simulink model "LV_grid"  (R2019b)
settings: Solver=VariableStepAuto  StartTime=0  StopTime=5.005  FixedStep=5e-4  RelTol=1e-3
model workspace (MAT data in the model file):
  P2_1 = 3450
libraries: powerlib x373, powerlib_meascontrol x37
(part 4 of 5)

== system LV_grid/L2/L1 ==
  Pi Section Line : powerlib/Elements/Pi Section Line  LConnTagsString=__new0  RConnTagsString=__new0  Frequency=50  Resistance=0.274  Inductance=0.073  Capacitance=12.74e-9  Length=0.0025  PiSections=1  Measurements=None
      settings: AttributesFormatString=\n  SourceProductName=Simscape Electrical  SourceProductBaseCode=PS
  Three-Phase PI Section Line : powerlib/Elements/Three-Phase PI Section Line  LConnTagsString=a|b|c  RConnTagsString=A|B|C  Frequency=50  Resistances=[ 0.274 0.959]  Inductances=[ 0.073 0.079]  Capacitances=[12.74e-9 7.751e-9]  Length=0.0025
      settings: SourceProductName=Simscape Electrical
  A : PMIOPort  Side=Left
  B : PMIOPort  Port=2  Side=Left
  C : PMIOPort  Port=3  Side=Left
  N : PMIOPort  Port=4  Side=Left
  a : PMIOPort  Port=5  Side=Right
  b : PMIOPort  Port=6  Side=Right
  c : PMIOPort  Port=7  Side=Right
  n : PMIOPort  Port=8  Side=Right
  connections:
  Pi Section Line/LConn1 -- N/RConn1
  Pi Section Line/RConn1 -- n/RConn1
  C/RConn1 -- Three-Phase PI Section Line/LConn3
  B/RConn1 -- Three-Phase PI Section Line/LConn2
  A/RConn1 -- Three-Phase PI Section Line/LConn1
  Three-Phase PI Section Line/RConn3 -- c/RConn1
  Three-Phase PI Section Line/RConn2 -- b/RConn1
  Three-Phase PI Section Line/RConn1 -- a/RConn1

== system LV_grid/L20/L1 ==
  Pi Section Line : powerlib/Elements/Pi Section Line  LConnTagsString=__new0  RConnTagsString=__new0  Frequency=50  Resistance=0.274  Inductance=0.073  Capacitance=12.74e-9  Length=0.0025  PiSections=1  Measurements=None
      settings: AttributesFormatString=\n  SourceProductName=Simscape Electrical  SourceProductBaseCode=PS
  Three-Phase PI Section Line : powerlib/Elements/Three-Phase PI Section Line  LConnTagsString=a|b|c  RConnTagsString=A|B|C  Frequency=50  Resistances=[ 0.274 0.959]  Inductances=[ 0.073 0.079]  Capacitances=[12.74e-9 7.751e-9]  Length=0.0025
      settings: SourceProductName=Simscape Electrical
  A : PMIOPort  Side=Left
  B : PMIOPort  Port=2  Side=Left
  C : PMIOPort  Port=3  Side=Left
  N : PMIOPort  Port=4  Side=Left
  a : PMIOPort  Port=5  Side=Right
  b : PMIOPort  Port=6  Side=Right
  c : PMIOPort  Port=7  Side=Right
  n : PMIOPort  Port=8  Side=Right
  connections:
  Pi Section Line/LConn1 -- N/RConn1
  Pi Section Line/RConn1 -- n/RConn1
  C/RConn1 -- Three-Phase PI Section Line/LConn3
  B/RConn1 -- Three-Phase PI Section Line/LConn2
  A/RConn1 -- Three-Phase PI Section Line/LConn1
  Three-Phase PI Section Line/RConn3 -- c/RConn1
  Three-Phase PI Section Line/RConn2 -- b/RConn1
  Three-Phase PI Section Line/RConn1 -- a/RConn1

== system LV_grid/L20/L2 ==
  Pi Section Line : powerlib/Elements/Pi Section Line  LConnTagsString=__new0  RConnTagsString=__new0  Frequency=50  Resistance=0.274  Inductance=0.073  Capacitance=12.74e-9  Length=0.0025  PiSections=1  Measurements=None
      settings: AttributesFormatString=\n  SourceProductName=Simscape Electrical  SourceProductBaseCode=PS
  Three-Phase PI Section Line : powerlib/Elements/Three-Phase PI Section Line  LConnTagsString=a|b|c  RConnTagsString=A|B|C  Frequency=50  Resistances=[ 0.274 0.959]  Inductances=[ 0.073 0.079]  Capacitances=[12.74e-9 7.751e-9]  Length=0.0025
      settings: SourceProductName=Simscape Electrical
  A : PMIOPort  Side=Left
  B : PMIOPort  Port=2  Side=Left
  C : PMIOPort  Port=3  Side=Left
  N : PMIOPort  Port=4  Side=Left
  a : PMIOPort  Port=5  Side=Right
  b : PMIOPort  Port=6  Side=Right
  c : PMIOPort  Port=7  Side=Right
  n : PMIOPort  Port=8  Side=Right
  connections:
  Pi Section Line/LConn1 -- N/RConn1
  Pi Section Line/RConn1 -- n/RConn1
  C/RConn1 -- Three-Phase PI Section Line/LConn3
  B/RConn1 -- Three-Phase PI Section Line/LConn2
  A/RConn1 -- Three-Phase PI Section Line/LConn1
  Three-Phase PI Section Line/RConn3 -- c/RConn1
  Three-Phase PI Section Line/RConn2 -- b/RConn1
  Three-Phase PI Section Line/RConn1 -- a/RConn1

== system LV_grid/L20/L3 ==
  Pi Section Line : powerlib/Elements/Pi Section Line  LConnTagsString=__new0  RConnTagsString=__new0  Frequency=50  Resistance=0.274  Inductance=0.073  Capacitance=12.74e-9  Length=0.0025  PiSections=1  Measurements=None
      settings: AttributesFormatString=\n  SourceProductName=Simscape Electrical  SourceProductBaseCode=PS
  Three-Phase PI Section Line : powerlib/Elements/Three-Phase PI Section Line  LConnTagsString=a|b|c  RConnTagsString=A|B|C  Frequency=50  Resistances=[ 0.274 0.959]  Inductances=[ 0.073 0.079]  Capacitances=[12.74e-9 7.751e-9]  Length=0.0025
      settings: SourceProductName=Simscape Electrical
  A : PMIOPort  Side=Left
  B : PMIOPort  Port=2  Side=Left
  C : PMIOPort  Port=3  Side=Left
  N : PMIOPort  Port=4  Side=Left
  a : PMIOPort  Port=5  Side=Right
  b : PMIOPort  Port=6  Side=Right
  c : PMIOPort  Port=7  Side=Right
  n : PMIOPort  Port=8  Side=Right
  connections:
  Pi Section Line/LConn1 -- N/RConn1
  Pi Section Line/RConn1 -- n/RConn1
  C/RConn1 -- Three-Phase PI Section Line/LConn3
  B/RConn1 -- Three-Phase PI Section Line/LConn2
  A/RConn1 -- Three-Phase PI Section Line/LConn1
  Three-Phase PI Section Line/RConn3 -- c/RConn1
  Three-Phase PI Section Line/RConn2 -- b/RConn1
  Three-Phase PI Section Line/RConn1 -- a/RConn1

== system LV_grid/L21/L1 ==
  Pi Section Line : powerlib/Elements/Pi Section Line  LConnTagsString=__new0  RConnTagsString=__new0  Frequency=50  Resistance=0.274  Inductance=0.073  Capacitance=12.74e-9  Length=0.0025  PiSections=1  Measurements=None
      settings: AttributesFormatString=\n  SourceProductName=Simscape Electrical  SourceProductBaseCode=PS
  Three-Phase PI Section Line : powerlib/Elements/Three-Phase PI Section Line  LConnTagsString=a|b|c  RConnTagsString=A|B|C  Frequency=50  Resistances=[ 0.274 0.959]  Inductances=[ 0.073 0.079]  Capacitances=[12.74e-9 7.751e-9]  Length=0.0025
      settings: SourceProductName=Simscape Electrical
  A : PMIOPort  Side=Left
  B : PMIOPort  Port=2  Side=Left
  C : PMIOPort  Port=3  Side=Left
  N : PMIOPort  Port=4  Side=Left
  a : PMIOPort  Port=5  Side=Right
  b : PMIOPort  Port=6  Side=Right
  c : PMIOPort  Port=7  Side=Right
  n : PMIOPort  Port=8  Side=Right
  connections:
  Pi Section Line/LConn1 -- N/RConn1
  Pi Section Line/RConn1 -- n/RConn1
  C/RConn1 -- Three-Phase PI Section Line/LConn3
  B/RConn1 -- Three-Phase PI Section Line/LConn2
  A/RConn1 -- Three-Phase PI Section Line/LConn1
  Three-Phase PI Section Line/RConn3 -- c/RConn1
  Three-Phase PI Section Line/RConn2 -- b/RConn1
  Three-Phase PI Section Line/RConn1 -- a/RConn1

== system LV_grid/L21/L2 ==
  Pi Section Line : powerlib/Elements/Pi Section Line  LConnTagsString=__new0  RConnTagsString=__new0  Frequency=50  Resistance=0.274  Inductance=0.073  Capacitance=12.74e-9  Length=0.0025  PiSections=1  Measurements=None
      settings: AttributesFormatString=\n  SourceProductName=Simscape Electrical  SourceProductBaseCode=PS
  Three-Phase PI Section Line : powerlib/Elements/Three-Phase PI Section Line  LConnTagsString=a|b|c  RConnTagsString=A|B|C  Frequency=50  Resistances=[ 0.274 0.959]  Inductances=[ 0.073 0.079]  Capacitances=[12.74e-9 7.751e-9]  Length=0.0025
      settings: SourceProductName=Simscape Electrical
  A : PMIOPort  Side=Left
  B : PMIOPort  Port=2  Side=Left
  C : PMIOPort  Port=3  Side=Left
  N : PMIOPort  Port=4  Side=Left
  a : PMIOPort  Port=5  Side=Right
  b : PMIOPort  Port=6  Side=Right
  c : PMIOPort  Port=7  Side=Right
  n : PMIOPort  Port=8  Side=Right
  connections:
  Pi Section Line/LConn1 -- N/RConn1
  Pi Section Line/RConn1 -- n/RConn1
  C/RConn1 -- Three-Phase PI Section Line/LConn3
  B/RConn1 -- Three-Phase PI Section Line/LConn2
  A/RConn1 -- Three-Phase PI Section Line/LConn1
  Three-Phase PI Section Line/RConn3 -- c/RConn1
  Three-Phase PI Section Line/RConn2 -- b/RConn1
  Three-Phase PI Section Line/RConn1 -- a/RConn1

== system LV_grid/L21/L3 ==
  Pi Section Line : powerlib/Elements/Pi Section Line  LConnTagsString=__new0  RConnTagsString=__new0  Frequency=50  Resistance=0.274  Inductance=0.073  Capacitance=12.74e-9  Length=0.0025  PiSections=1  Measurements=None
      settings: AttributesFormatString=\n  SourceProductName=Simscape Electrical  SourceProductBaseCode=PS
  Three-Phase PI Section Line : powerlib/Elements/Three-Phase PI Section Line  LConnTagsString=a|b|c  RConnTagsString=A|B|C  Frequency=50  Resistances=[ 0.274 0.959]  Inductances=[ 0.073 0.079]  Capacitances=[12.74e-9 7.751e-9]  Length=0.0025
      settings: SourceProductName=Simscape Electrical
  A : PMIOPort  Side=Left
  B : PMIOPort  Port=2  Side=Left
  C : PMIOPort  Port=3  Side=Left
  N : PMIOPort  Port=4  Side=Left
  a : PMIOPort  Port=5  Side=Right
  b : PMIOPort  Port=6  Side=Right
  c : PMIOPort  Port=7  Side=Right
  n : PMIOPort  Port=8  Side=Right
  connections:
  Pi Section Line/LConn1 -- N/RConn1
  Pi Section Line/RConn1 -- n/RConn1
  C/RConn1 -- Three-Phase PI Section Line/LConn3
  B/RConn1 -- Three-Phase PI Section Line/LConn2
  A/RConn1 -- Three-Phase PI Section Line/LConn1
  Three-Phase PI Section Line/RConn3 -- c/RConn1
  Three-Phase PI Section Line/RConn2 -- b/RConn1
  Three-Phase PI Section Line/RConn1 -- a/RConn1

== system LV_grid/L21/L4 ==
  Pi Section Line : powerlib/Elements/Pi Section Line  LConnTagsString=__new0  RConnTagsString=__new0  Frequency=50  Resistance=0.274  Inductance=0.073  Capacitance=12.74e-9  Length=0.0025  PiSections=1  Measurements=None
      settings: AttributesFormatString=\n  SourceProductName=Simscape Electrical  SourceProductBaseCode=PS
  Three-Phase PI Section Line : powerlib/Elements/Three-Phase PI Section Line  LConnTagsString=a|b|c  RConnTagsString=A|B|C  Frequency=50  Resistances=[ 0.274 0.959]  Inductances=[ 0.073 0.079]  Capacitances=[12.74e-9 7.751e-9]  Length=0.0025
      settings: SourceProductName=Simscape Electrical
  A : PMIOPort  Side=Left
  B : PMIOPort  Port=2  Side=Left
  C : PMIOPort  Port=3  Side=Left
  N : PMIOPort  Port=4  Side=Left
  a : PMIOPort  Port=5  Side=Right
  b : PMIOPort  Port=6  Side=Right
  c : PMIOPort  Port=7  Side=Right
  n : PMIOPort  Port=8  Side=Right
  connections:
  Pi Section Line/LConn1 -- N/RConn1
  Pi Section Line/RConn1 -- n/RConn1
  C/RConn1 -- Three-Phase PI Section Line/LConn3
  B/RConn1 -- Three-Phase PI Section Line/LConn2
  A/RConn1 -- Three-Phase PI Section Line/LConn1
  Three-Phase PI Section Line/RConn3 -- c/RConn1
  Three-Phase PI Section Line/RConn2 -- b/RConn1
  Three-Phase PI Section Line/RConn1 -- a/RConn1

== system LV_grid/L21/L5 ==
  Pi Section Line : powerlib/Elements/Pi Section Line  LConnTagsString=__new0  RConnTagsString=__new0  Frequency=50  Resistance=0.274  Inductance=0.073  Capacitance=12.74e-9  Length=0.0025  PiSections=1  Measurements=None
      settings: AttributesFormatString=\n  SourceProductName=Simscape Electrical  SourceProductBaseCode=PS
  Three-Phase PI Section Line : powerlib/Elements/Three-Phase PI Section Line  LConnTagsString=a|b|c  RConnTagsString=A|B|C  Frequency=50  Resistances=[ 0.274 0.959]  Inductances=[ 0.073 0.079]  Capacitances=[12.74e-9 7.751e-9]  Length=0.0025
      settings: SourceProductName=Simscape Electrical
  A : PMIOPort  Side=Left
  B : PMIOPort  Port=2  Side=Left
  C : PMIOPort  Port=3  Side=Left
  N : PMIOPort  Port=4  Side=Left
  a : PMIOPort  Port=5  Side=Right
  b : PMIOPort  Port=6  Side=Right
  c : PMIOPort  Port=7  Side=Right
  n : PMIOPort  Port=8  Side=Right
  connections:
  Pi Section Line/LConn1 -- N/RConn1
  Pi Section Line/RConn1 -- n/RConn1
  C/RConn1 -- Three-Phase PI Section Line/LConn3
  B/RConn1 -- Three-Phase PI Section Line/LConn2
  A/RConn1 -- Three-Phase PI Section Line/LConn1
  Three-Phase PI Section Line/RConn3 -- c/RConn1
  Three-Phase PI Section Line/RConn2 -- b/RConn1
  Three-Phase PI Section Line/RConn1 -- a/RConn1

== system LV_grid/L22/L1 ==
  Pi Section Line : powerlib/Elements/Pi Section Line  LConnTagsString=__new0  RConnTagsString=__new0  Frequency=50  Resistance=0.274  Inductance=0.073  Capacitance=12.74e-9  Length=0.0025  PiSections=1  Measurements=None
      settings: AttributesFormatString=\n  SourceProductName=Simscape Electrical  SourceProductBaseCode=PS
  Three-Phase PI Section Line : powerlib/Elements/Three-Phase PI Section Line  LConnTagsString=a|b|c  RConnTagsString=A|B|C  Frequency=50  Resistances=[ 0.274 0.959]  Inductances=[ 0.073 0.079]  Capacitances=[12.74e-9 7.751e-9]  Length=0.0025
      settings: SourceProductName=Simscape Electrical
  A : PMIOPort  Side=Left
  B : PMIOPort  Port=2  Side=Left
  C : PMIOPort  Port=3  Side=Left
  N : PMIOPort  Port=4  Side=Left
  a : PMIOPort  Port=5  Side=Right
  b : PMIOPort  Port=6  Side=Right
  c : PMIOPort  Port=7  Side=Right
  n : PMIOPort  Port=8  Side=Right
  connections:
  Pi Section Line/LConn1 -- N/RConn1
  Pi Section Line/RConn1 -- n/RConn1
  C/RConn1 -- Three-Phase PI Section Line/LConn3
  B/RConn1 -- Three-Phase PI Section Line/LConn2
  A/RConn1 -- Three-Phase PI Section Line/LConn1
  Three-Phase PI Section Line/RConn3 -- c/RConn1
  Three-Phase PI Section Line/RConn2 -- b/RConn1
  Three-Phase PI Section Line/RConn1 -- a/RConn1

== system LV_grid/L22/L2 ==
  Pi Section Line : powerlib/Elements/Pi Section Line  LConnTagsString=__new0  RConnTagsString=__new0  Frequency=50  Resistance=0.274  Inductance=0.073  Capacitance=12.74e-9  Length=0.0025  PiSections=1  Measurements=None
      settings: AttributesFormatString=\n  SourceProductName=Simscape Electrical  SourceProductBaseCode=PS
  Three-Phase PI Section Line : powerlib/Elements/Three-Phase PI Section Line  LConnTagsString=a|b|c  RConnTagsString=A|B|C  Frequency=50  Resistances=[ 0.274 0.959]  Inductances=[ 0.073 0.079]  Capacitances=[12.74e-9 7.751e-9]  Length=0.0025
      settings: SourceProductName=Simscape Electrical
  A : PMIOPort  Side=Left
  B : PMIOPort  Port=2  Side=Left
  C : PMIOPort  Port=3  Side=Left
  N : PMIOPort  Port=4  Side=Left
  a : PMIOPort  Port=5  Side=Right
  b : PMIOPort  Port=6  Side=Right
  c : PMIOPort  Port=7  Side=Right
  n : PMIOPort  Port=8  Side=Right
  connections:
  Pi Section Line/LConn1 -- N/RConn1
  Pi Section Line/RConn1 -- n/RConn1
  C/RConn1 -- Three-Phase PI Section Line/LConn3
  B/RConn1 -- Three-Phase PI Section Line/LConn2
  A/RConn1 -- Three-Phase PI Section Line/LConn1
  Three-Phase PI Section Line/RConn3 -- c/RConn1
  Three-Phase PI Section Line/RConn2 -- b/RConn1
  Three-Phase PI Section Line/RConn1 -- a/RConn1

== system LV_grid/L23/L1 ==
  Pi Section Line : powerlib/Elements/Pi Section Line  LConnTagsString=__new0  RConnTagsString=__new0  Frequency=50  Resistance=0.274  Inductance=0.073  Capacitance=12.74e-9  Length=0.0025  PiSections=1  Measurements=None
      settings: AttributesFormatString=\n  SourceProductName=Simscape Electrical  SourceProductBaseCode=PS
  Three-Phase PI Section Line : powerlib/Elements/Three-Phase PI Section Line  LConnTagsString=a|b|c  RConnTagsString=A|B|C  Frequency=50  Resistances=[ 0.274 0.959]  Inductances=[ 0.073 0.079]  Capacitances=[12.74e-9 7.751e-9]  Length=0.0025
      settings: SourceProductName=Simscape Electrical
  A : PMIOPort  Side=Left
  B : PMIOPort  Port=2  Side=Left
  C : PMIOPort  Port=3  Side=Left
  N : PMIOPort  Port=4  Side=Left
  a : PMIOPort  Port=5  Side=Right
  b : PMIOPort  Port=6  Side=Right
  c : PMIOPort  Port=7  Side=Right
  n : PMIOPort  Port=8  Side=Right
  connections:
  Pi Section Line/LConn1 -- N/RConn1
  Pi Section Line/RConn1 -- n/RConn1
  C/RConn1 -- Three-Phase PI Section Line/LConn3
  B/RConn1 -- Three-Phase PI Section Line/LConn2
  A/RConn1 -- Three-Phase PI Section Line/LConn1
  Three-Phase PI Section Line/RConn3 -- c/RConn1
  Three-Phase PI Section Line/RConn2 -- b/RConn1
  Three-Phase PI Section Line/RConn1 -- a/RConn1

== system LV_grid/L23/L2 ==
  Pi Section Line : powerlib/Elements/Pi Section Line  LConnTagsString=__new0  RConnTagsString=__new0  Frequency=50  Resistance=0.274  Inductance=0.073  Capacitance=12.74e-9  Length=0.0025  PiSections=1  Measurements=None
      settings: AttributesFormatString=\n  SourceProductName=Simscape Electrical  SourceProductBaseCode=PS
  Three-Phase PI Section Line : powerlib/Elements/Three-Phase PI Section Line  LConnTagsString=a|b|c  RConnTagsString=A|B|C  Frequency=50  Resistances=[ 0.274 0.959]  Inductances=[ 0.073 0.079]  Capacitances=[12.74e-9 7.751e-9]  Length=0.0025
      settings: SourceProductName=Simscape Electrical
  A : PMIOPort  Side=Left
  B : PMIOPort  Port=2  Side=Left
  C : PMIOPort  Port=3  Side=Left
  N : PMIOPort  Port=4  Side=Left
  a : PMIOPort  Port=5  Side=Right
  b : PMIOPort  Port=6  Side=Right
  c : PMIOPort  Port=7  Side=Right
  n : PMIOPort  Port=8  Side=Right
  connections:
  Pi Section Line/LConn1 -- N/RConn1
  Pi Section Line/RConn1 -- n/RConn1
  C/RConn1 -- Three-Phase PI Section Line/LConn3
  B/RConn1 -- Three-Phase PI Section Line/LConn2
  A/RConn1 -- Three-Phase PI Section Line/LConn1
  Three-Phase PI Section Line/RConn3 -- c/RConn1
  Three-Phase PI Section Line/RConn2 -- b/RConn1
  Three-Phase PI Section Line/RConn1 -- a/RConn1

== system LV_grid/L23/L3 ==
  Pi Section Line : powerlib/Elements/Pi Section Line  LConnTagsString=__new0  RConnTagsString=__new0  Frequency=50  Resistance=0.274  Inductance=0.073  Capacitance=12.74e-9  Length=0.0025  PiSections=1  Measurements=None
      settings: AttributesFormatString=\n  SourceProductName=Simscape Electrical  SourceProductBaseCode=PS
  Three-Phase PI Section Line : powerlib/Elements/Three-Phase PI Section Line  LConnTagsString=a|b|c  RConnTagsString=A|B|C  Frequency=50  Resistances=[ 0.274 0.959]  Inductances=[ 0.073 0.079]  Capacitances=[12.74e-9 7.751e-9]  Length=0.0025
      settings: SourceProductName=Simscape Electrical
  A : PMIOPort  Side=Left
  B : PMIOPort  Port=2  Side=Left
  C : PMIOPort  Port=3  Side=Left
  N : PMIOPort  Port=4  Side=Left
  a : PMIOPort  Port=5  Side=Right
  b : PMIOPort  Port=6  Side=Right
  c : PMIOPort  Port=7  Side=Right
  n : PMIOPort  Port=8  Side=Right
  connections:
  Pi Section Line/LConn1 -- N/RConn1
  Pi Section Line/RConn1 -- n/RConn1
  C/RConn1 -- Three-Phase PI Section Line/LConn3
  B/RConn1 -- Three-Phase PI Section Line/LConn2
  A/RConn1 -- Three-Phase PI Section Line/LConn1
  Three-Phase PI Section Line/RConn3 -- c/RConn1
  Three-Phase PI Section Line/RConn2 -- b/RConn1
  Three-Phase PI Section Line/RConn1 -- a/RConn1

== system LV_grid/L23/L4 ==
  Pi Section Line : powerlib/Elements/Pi Section Line  LConnTagsString=__new0  RConnTagsString=__new0  Frequency=50  Resistance=0.274  Inductance=0.073  Capacitance=12.74e-9  Length=0.0025  PiSections=1  Measurements=None
      settings: AttributesFormatString=\n  SourceProductName=Simscape Electrical  SourceProductBaseCode=PS
  Three-Phase PI Section Line : powerlib/Elements/Three-Phase PI Section Line  LConnTagsString=a|b|c  RConnTagsString=A|B|C  Frequency=50  Resistances=[ 0.274 0.959]  Inductances=[ 0.073 0.079]  Capacitances=[12.74e-9 7.751e-9]  Length=0.0025
      settings: SourceProductName=Simscape Electrical
  A : PMIOPort  Side=Left
  B : PMIOPort  Port=2  Side=Left
  C : PMIOPort  Port=3  Side=Left
  N : PMIOPort  Port=4  Side=Left
  a : PMIOPort  Port=5  Side=Right
  b : PMIOPort  Port=6  Side=Right
  c : PMIOPort  Port=7  Side=Right
  n : PMIOPort  Port=8  Side=Right
  connections:
  Pi Section Line/LConn1 -- N/RConn1
  Pi Section Line/RConn1 -- n/RConn1
  C/RConn1 -- Three-Phase PI Section Line/LConn3
  B/RConn1 -- Three-Phase PI Section Line/LConn2
  A/RConn1 -- Three-Phase PI Section Line/LConn1
  Three-Phase PI Section Line/RConn3 -- c/RConn1
  Three-Phase PI Section Line/RConn2 -- b/RConn1
  Three-Phase PI Section Line/RConn1 -- a/RConn1

== system LV_grid/L23/L5 ==
  Pi Section Line : powerlib/Elements/Pi Section Line  LConnTagsString=__new0  RConnTagsString=__new0  Frequency=50  Resistance=0.274  Inductance=0.073  Capacitance=12.74e-9  Length=0.0025  PiSections=1  Measurements=None
      settings: AttributesFormatString=\n  SourceProductName=Simscape Electrical  SourceProductBaseCode=PS
  Three-Phase PI Section Line : powerlib/Elements/Three-Phase PI Section Line  LConnTagsString=a|b|c  RConnTagsString=A|B|C  Frequency=50  Resistances=[ 0.274 0.959]  Inductances=[ 0.073 0.079]  Capacitances=[12.74e-9 7.751e-9]  Length=0.0025
      settings: SourceProductName=Simscape Electrical
  A : PMIOPort  Side=Left
  B : PMIOPort  Port=2  Side=Left
  C : PMIOPort  Port=3  Side=Left
  N : PMIOPort  Port=4  Side=Left
  a : PMIOPort  Port=5  Side=Right
  b : PMIOPort  Port=6  Side=Right
  c : PMIOPort  Port=7  Side=Right
  n : PMIOPort  Port=8  Side=Right
  connections:
  Pi Section Line/LConn1 -- N/RConn1
  Pi Section Line/RConn1 -- n/RConn1
  C/RConn1 -- Three-Phase PI Section Line/LConn3
  B/RConn1 -- Three-Phase PI Section Line/LConn2
  A/RConn1 -- Three-Phase PI Section Line/LConn1
  Three-Phase PI Section Line/RConn3 -- c/RConn1
  Three-Phase PI Section Line/RConn2 -- b/RConn1
  Three-Phase PI Section Line/RConn1 -- a/RConn1

== system LV_grid/L24/L1 ==
  Pi Section Line : powerlib/Elements/Pi Section Line  LConnTagsString=__new0  RConnTagsString=__new0  Frequency=50  Resistance=0.274  Inductance=0.073  Capacitance=12.74e-9  Length=0.0025  PiSections=1  Measurements=None
      settings: AttributesFormatString=\n  SourceProductName=Simscape Electrical  SourceProductBaseCode=PS
  Three-Phase PI Section Line : powerlib/Elements/Three-Phase PI Section Line  LConnTagsString=a|b|c  RConnTagsString=A|B|C  Frequency=50  Resistances=[ 0.274 0.959]  Inductances=[ 0.073 0.079]  Capacitances=[12.74e-9 7.751e-9]  Length=0.0025
      settings: SourceProductName=Simscape Electrical
  A : PMIOPort  Side=Left
  B : PMIOPort  Port=2  Side=Left
  C : PMIOPort  Port=3  Side=Left
  N : PMIOPort  Port=4  Side=Left
  a : PMIOPort  Port=5  Side=Right
  b : PMIOPort  Port=6  Side=Right
  c : PMIOPort  Port=7  Side=Right
  n : PMIOPort  Port=8  Side=Right
  connections:
  Pi Section Line/LConn1 -- N/RConn1
  Pi Section Line/RConn1 -- n/RConn1
  C/RConn1 -- Three-Phase PI Section Line/LConn3
  B/RConn1 -- Three-Phase PI Section Line/LConn2
  A/RConn1 -- Three-Phase PI Section Line/LConn1
  Three-Phase PI Section Line/RConn3 -- c/RConn1
  Three-Phase PI Section Line/RConn2 -- b/RConn1
  Three-Phase PI Section Line/RConn1 -- a/RConn1

== system LV_grid/L24/L2 ==
  Pi Section Line : powerlib/Elements/Pi Section Line  LConnTagsString=__new0  RConnTagsString=__new0  Frequency=50  Resistance=0.274  Inductance=0.073  Capacitance=12.74e-9  Length=0.0025  PiSections=1  Measurements=None
      settings: AttributesFormatString=\n  SourceProductName=Simscape Electrical  SourceProductBaseCode=PS
  Three-Phase PI Section Line : powerlib/Elements/Three-Phase PI Section Line  LConnTagsString=a|b|c  RConnTagsString=A|B|C  Frequency=50  Resistances=[ 0.274 0.959]  Inductances=[ 0.073 0.079]  Capacitances=[12.74e-9 7.751e-9]  Length=0.0025
      settings: SourceProductName=Simscape Electrical
  A : PMIOPort  Side=Left
  B : PMIOPort  Port=2  Side=Left
  C : PMIOPort  Port=3  Side=Left
  N : PMIOPort  Port=4  Side=Left
  a : PMIOPort  Port=5  Side=Right
  b : PMIOPort  Port=6  Side=Right
  c : PMIOPort  Port=7  Side=Right
  n : PMIOPort  Port=8  Side=Right
  connections:
  Pi Section Line/LConn1 -- N/RConn1
  Pi Section Line/RConn1 -- n/RConn1
  C/RConn1 -- Three-Phase PI Section Line/LConn3
  B/RConn1 -- Three-Phase PI Section Line/LConn2
  A/RConn1 -- Three-Phase PI Section Line/LConn1
  Three-Phase PI Section Line/RConn3 -- c/RConn1
  Three-Phase PI Section Line/RConn2 -- b/RConn1
  Three-Phase PI Section Line/RConn1 -- a/RConn1

== system LV_grid/L24/L3 ==
  Pi Section Line : powerlib/Elements/Pi Section Line  LConnTagsString=__new0  RConnTagsString=__new0  Frequency=50  Resistance=0.274  Inductance=0.073  Capacitance=12.74e-9  Length=0.0025  PiSections=1  Measurements=None
      settings: AttributesFormatString=\n  SourceProductName=Simscape Electrical  SourceProductBaseCode=PS
  Three-Phase PI Section Line : powerlib/Elements/Three-Phase PI Section Line  LConnTagsString=a|b|c  RConnTagsString=A|B|C  Frequency=50  Resistances=[ 0.274 0.959]  Inductances=[ 0.073 0.079]  Capacitances=[12.74e-9 7.751e-9]  Length=0.0025
      settings: SourceProductName=Simscape Electrical
  A : PMIOPort  Side=Left
  B : PMIOPort  Port=2  Side=Left
  C : PMIOPort  Port=3  Side=Left
  N : PMIOPort  Port=4  Side=Left
  a : PMIOPort  Port=5  Side=Right
  b : PMIOPort  Port=6  Side=Right
  c : PMIOPort  Port=7  Side=Right
  n : PMIOPort  Port=8  Side=Right
  connections:
  Pi Section Line/LConn1 -- N/RConn1
  Pi Section Line/RConn1 -- n/RConn1
  C/RConn1 -- Three-Phase PI Section Line/LConn3
  B/RConn1 -- Three-Phase PI Section Line/LConn2
  A/RConn1 -- Three-Phase PI Section Line/LConn1
  Three-Phase PI Section Line/RConn3 -- c/RConn1
  Three-Phase PI Section Line/RConn2 -- b/RConn1
  Three-Phase PI Section Line/RConn1 -- a/RConn1

== system LV_grid/L24/L4 ==
  Pi Section Line : powerlib/Elements/Pi Section Line  LConnTagsString=__new0  RConnTagsString=__new0  Frequency=50  Resistance=0.274  Inductance=0.073  Capacitance=12.74e-9  Length=0.0025  PiSections=1  Measurements=None
      settings: AttributesFormatString=\n  SourceProductName=Simscape Electrical  SourceProductBaseCode=PS
  Three-Phase PI Section Line : powerlib/Elements/Three-Phase PI Section Line  LConnTagsString=a|b|c  RConnTagsString=A|B|C  Frequency=50  Resistances=[ 0.274 0.959]  Inductances=[ 0.073 0.079]  Capacitances=[12.74e-9 7.751e-9]  Length=0.0025
      settings: SourceProductName=Simscape Electrical
  A : PMIOPort  Side=Left
  B : PMIOPort  Port=2  Side=Left
  C : PMIOPort  Port=3  Side=Left
  N : PMIOPort  Port=4  Side=Left
  a : PMIOPort  Port=5  Side=Right
  b : PMIOPort  Port=6  Side=Right
  c : PMIOPort  Port=7  Side=Right
  n : PMIOPort  Port=8  Side=Right
  connections:
  Pi Section Line/LConn1 -- N/RConn1
  Pi Section Line/RConn1 -- n/RConn1
  C/RConn1 -- Three-Phase PI Section Line/LConn3
  B/RConn1 -- Three-Phase PI Section Line/LConn2
  A/RConn1 -- Three-Phase PI Section Line/LConn1
  Three-Phase PI Section Line/RConn3 -- c/RConn1
  Three-Phase PI Section Line/RConn2 -- b/RConn1
  Three-Phase PI Section Line/RConn1 -- a/RConn1

== system LV_grid/L25/L1 ==
  Pi Section Line : powerlib/Elements/Pi Section Line  LConnTagsString=__new0  RConnTagsString=__new0  Frequency=50  Resistance=0.274  Inductance=0.073  Capacitance=12.74e-9  Length=0.0025  PiSections=1  Measurements=None
      settings: AttributesFormatString=\n  SourceProductName=Simscape Electrical  SourceProductBaseCode=PS
  Three-Phase PI Section Line : powerlib/Elements/Three-Phase PI Section Line  LConnTagsString=a|b|c  RConnTagsString=A|B|C  Frequency=50  Resistances=[ 0.274 0.959]  Inductances=[ 0.073 0.079]  Capacitances=[12.74e-9 7.751e-9]  Length=0.0025
      settings: SourceProductName=Simscape Electrical
  A : PMIOPort  Side=Left
  B : PMIOPort  Port=2  Side=Left
  C : PMIOPort  Port=3  Side=Left
  N : PMIOPort  Port=4  Side=Left
  a : PMIOPort  Port=5  Side=Right
  b : PMIOPort  Port=6  Side=Right
  c : PMIOPort  Port=7  Side=Right
  n : PMIOPort  Port=8  Side=Right
  connections:
  Pi Section Line/LConn1 -- N/RConn1
  Pi Section Line/RConn1 -- n/RConn1
  C/RConn1 -- Three-Phase PI Section Line/LConn3
  B/RConn1 -- Three-Phase PI Section Line/LConn2
  A/RConn1 -- Three-Phase PI Section Line/LConn1
  Three-Phase PI Section Line/RConn3 -- c/RConn1
  Three-Phase PI Section Line/RConn2 -- b/RConn1
  Three-Phase PI Section Line/RConn1 -- a/RConn1

== system LV_grid/L25/L2 ==
  Pi Section Line : powerlib/Elements/Pi Section Line  LConnTagsString=__new0  RConnTagsString=__new0  Frequency=50  Resistance=0.274  Inductance=0.073  Capacitance=12.74e-9  Length=0.0025  PiSections=1  Measurements=None
      settings: AttributesFormatString=\n  SourceProductName=Simscape Electrical  SourceProductBaseCode=PS
  Three-Phase PI Section Line : powerlib/Elements/Three-Phase PI Section Line  LConnTagsString=a|b|c  RConnTagsString=A|B|C  Frequency=50  Resistances=[ 0.274 0.959]  Inductances=[ 0.073 0.079]  Capacitances=[12.74e-9 7.751e-9]  Length=0.0025
      settings: SourceProductName=Simscape Electrical
  A : PMIOPort  Side=Left
  B : PMIOPort  Port=2  Side=Left
  C : PMIOPort  Port=3  Side=Left
  N : PMIOPort  Port=4  Side=Left
  a : PMIOPort  Port=5  Side=Right
  b : PMIOPort  Port=6  Side=Right
  c : PMIOPort  Port=7  Side=Right
  n : PMIOPort  Port=8  Side=Right
  connections:
  Pi Section Line/LConn1 -- N/RConn1
  Pi Section Line/RConn1 -- n/RConn1
  C/RConn1 -- Three-Phase PI Section Line/LConn3
  B/RConn1 -- Three-Phase PI Section Line/LConn2
  A/RConn1 -- Three-Phase PI Section Line/LConn1
  Three-Phase PI Section Line/RConn3 -- c/RConn1
  Three-Phase PI Section Line/RConn2 -- b/RConn1
  Three-Phase PI Section Line/RConn1 -- a/RConn1

== system LV_grid/L25/L3 ==
  Pi Section Line : powerlib/Elements/Pi Section Line  LConnTagsString=__new0  RConnTagsString=__new0  Frequency=50  Resistance=0.274  Inductance=0.073  Capacitance=12.74e-9  Length=0.0025  PiSections=1  Measurements=None
      settings: AttributesFormatString=\n  SourceProductName=Simscape Electrical  SourceProductBaseCode=PS
  Three-Phase PI Section Line : powerlib/Elements/Three-Phase PI Section Line  LConnTagsString=a|b|c  RConnTagsString=A|B|C  Frequency=50  Resistances=[ 0.274 0.959]  Inductances=[ 0.073 0.079]  Capacitances=[12.74e-9 7.751e-9]  Length=0.0025
      settings: SourceProductName=Simscape Electrical
  A : PMIOPort  Side=Left
  B : PMIOPort  Port=2  Side=Left
  C : PMIOPort  Port=3  Side=Left
  N : PMIOPort  Port=4  Side=Left
  a : PMIOPort  Port=5  Side=Right
  b : PMIOPort  Port=6  Side=Right
  c : PMIOPort  Port=7  Side=Right
  n : PMIOPort  Port=8  Side=Right
  connections:
  Pi Section Line/LConn1 -- N/RConn1
  Pi Section Line/RConn1 -- n/RConn1
  C/RConn1 -- Three-Phase PI Section Line/LConn3
  B/RConn1 -- Three-Phase PI Section Line/LConn2
  A/RConn1 -- Three-Phase PI Section Line/LConn1
  Three-Phase PI Section Line/RConn3 -- c/RConn1
  Three-Phase PI Section Line/RConn2 -- b/RConn1
  Three-Phase PI Section Line/RConn1 -- a/RConn1

== system LV_grid/L25/L4 ==
  Pi Section Line : powerlib/Elements/Pi Section Line  LConnTagsString=__new0  RConnTagsString=__new0  Frequency=50  Resistance=0.274  Inductance=0.073  Capacitance=12.74e-9  Length=0.0025  PiSections=1  Measurements=None
      settings: AttributesFormatString=\n  SourceProductName=Simscape Electrical  SourceProductBaseCode=PS
  Three-Phase PI Section Line : powerlib/Elements/Three-Phase PI Section Line  LConnTagsString=a|b|c  RConnTagsString=A|B|C  Frequency=50  Resistances=[ 0.274 0.959]  Inductances=[ 0.073 0.079]  Capacitances=[12.74e-9 7.751e-9]  Length=0.0025
      settings: SourceProductName=Simscape Electrical
  A : PMIOPort  Side=Left
  B : PMIOPort  Port=2  Side=Left
  C : PMIOPort  Port=3  Side=Left
  N : PMIOPort  Port=4  Side=Left
  a : PMIOPort  Port=5  Side=Right
  b : PMIOPort  Port=6  Side=Right
  c : PMIOPort  Port=7  Side=Right
  n : PMIOPort  Port=8  Side=Right
  connections:
  Pi Section Line/LConn1 -- N/RConn1
  Pi Section Line/RConn1 -- n/RConn1
  C/RConn1 -- Three-Phase PI Section Line/LConn3
  B/RConn1 -- Three-Phase PI Section Line/LConn2
  A/RConn1 -- Three-Phase PI Section Line/LConn1
  Three-Phase PI Section Line/RConn3 -- c/RConn1
  Three-Phase PI Section Line/RConn2 -- b/RConn1
  Three-Phase PI Section Line/RConn1 -- a/RConn1

== system LV_grid/L26/L1 ==
  Pi Section Line : powerlib/Elements/Pi Section Line  LConnTagsString=__new0  RConnTagsString=__new0  Frequency=50  Resistance=0.274  Inductance=0.073  Capacitance=12.74e-9  Length=0.0025  PiSections=1  Measurements=None
      settings: AttributesFormatString=\n  SourceProductName=Simscape Electrical  SourceProductBaseCode=PS
  Three-Phase PI Section Line : powerlib/Elements/Three-Phase PI Section Line  LConnTagsString=a|b|c  RConnTagsString=A|B|C  Frequency=50  Resistances=[ 0.274 0.959]  Inductances=[ 0.073 0.079]  Capacitances=[12.74e-9 7.751e-9]  Length=0.0025
      settings: SourceProductName=Simscape Electrical
  A : PMIOPort  Side=Left
  B : PMIOPort  Port=2  Side=Left
  C : PMIOPort  Port=3  Side=Left
  N : PMIOPort  Port=4  Side=Left
  a : PMIOPort  Port=5  Side=Right
  b : PMIOPort  Port=6  Side=Right
  c : PMIOPort  Port=7  Side=Right
  n : PMIOPort  Port=8  Side=Right
  connections:
  Pi Section Line/LConn1 -- N/RConn1
  Pi Section Line/RConn1 -- n/RConn1
  C/RConn1 -- Three-Phase PI Section Line/LConn3
  B/RConn1 -- Three-Phase PI Section Line/LConn2
  A/RConn1 -- Three-Phase PI Section Line/LConn1
  Three-Phase PI Section Line/RConn3 -- c/RConn1
  Three-Phase PI Section Line/RConn2 -- b/RConn1
  Three-Phase PI Section Line/RConn1 -- a/RConn1

== system LV_grid/L26/L2 ==
  Pi Section Line : powerlib/Elements/Pi Section Line  LConnTagsString=__new0  RConnTagsString=__new0  Frequency=50  Resistance=0.274  Inductance=0.073  Capacitance=12.74e-9  Length=0.0025  PiSections=1  Measurements=None
      settings: AttributesFormatString=\n  SourceProductName=Simscape Electrical  SourceProductBaseCode=PS
  Three-Phase PI Section Line : powerlib/Elements/Three-Phase PI Section Line  LConnTagsString=a|b|c  RConnTagsString=A|B|C  Frequency=50  Resistances=[ 0.274 0.959]  Inductances=[ 0.073 0.079]  Capacitances=[12.74e-9 7.751e-9]  Length=0.0025
      settings: SourceProductName=Simscape Electrical
  A : PMIOPort  Side=Left
  B : PMIOPort  Port=2  Side=Left
  C : PMIOPort  Port=3  Side=Left
  N : PMIOPort  Port=4  Side=Left
  a : PMIOPort  Port=5  Side=Right
  b : PMIOPort  Port=6  Side=Right
  c : PMIOPort  Port=7  Side=Right
  n : PMIOPort  Port=8  Side=Right
  connections:
  Pi Section Line/LConn1 -- N/RConn1
  Pi Section Line/RConn1 -- n/RConn1
  C/RConn1 -- Three-Phase PI Section Line/LConn3
  B/RConn1 -- Three-Phase PI Section Line/LConn2
  A/RConn1 -- Three-Phase PI Section Line/LConn1
  Three-Phase PI Section Line/RConn3 -- c/RConn1
  Three-Phase PI Section Line/RConn2 -- b/RConn1
  Three-Phase PI Section Line/RConn1 -- a/RConn1

== system LV_grid/L27/L1 ==
  Pi Section Line : powerlib/Elements/Pi Section Line  LConnTagsString=__new0  RConnTagsString=__new0  Frequency=50  Resistance=0.274  Inductance=0.073  Capacitance=12.74e-9  Length=0.0025  PiSections=1  Measurements=None
      settings: AttributesFormatString=\n  SourceProductName=Simscape Electrical  SourceProductBaseCode=PS
  Three-Phase PI Section Line : powerlib/Elements/Three-Phase PI Section Line  LConnTagsString=a|b|c  RConnTagsString=A|B|C  Frequency=50  Resistances=[ 0.274 0.959]  Inductances=[ 0.073 0.079]  Capacitances=[12.74e-9 7.751e-9]  Length=0.0025
      settings: SourceProductName=Simscape Electrical
  A : PMIOPort  Side=Left
  B : PMIOPort  Port=2  Side=Left
  C : PMIOPort  Port=3  Side=Left
  N : PMIOPort  Port=4  Side=Left
  a : PMIOPort  Port=5  Side=Right
  b : PMIOPort  Port=6  Side=Right
  c : PMIOPort  Port=7  Side=Right
  n : PMIOPort  Port=8  Side=Right
  connections:
  Pi Section Line/LConn1 -- N/RConn1
  Pi Section Line/RConn1 -- n/RConn1
  C/RConn1 -- Three-Phase PI Section Line/LConn3
  B/RConn1 -- Three-Phase PI Section Line/LConn2
  A/RConn1 -- Three-Phase PI Section Line/LConn1
  Three-Phase PI Section Line/RConn3 -- c/RConn1
  Three-Phase PI Section Line/RConn2 -- b/RConn1
  Three-Phase PI Section Line/RConn1 -- a/RConn1

== system LV_grid/L27/L2 ==
  Pi Section Line : powerlib/Elements/Pi Section Line  LConnTagsString=__new0  RConnTagsString=__new0  Frequency=50  Resistance=0.274  Inductance=0.073  Capacitance=12.74e-9  Length=0.0025  PiSections=1  Measurements=None
      settings: AttributesFormatString=\n  SourceProductName=Simscape Electrical  SourceProductBaseCode=PS
  Three-Phase PI Section Line : powerlib/Elements/Three-Phase PI Section Line  LConnTagsString=a|b|c  RConnTagsString=A|B|C  Frequency=50  Resistances=[ 0.274 0.959]  Inductances=[ 0.073 0.079]  Capacitances=[12.74e-9 7.751e-9]  Length=0.0025
      settings: SourceProductName=Simscape Electrical
  A : PMIOPort  Side=Left
  B : PMIOPort  Port=2  Side=Left
  C : PMIOPort  Port=3  Side=Left
  N : PMIOPort  Port=4  Side=Left
  a : PMIOPort  Port=5  Side=Right
  b : PMIOPort  Port=6  Side=Right
  c : PMIOPort  Port=7  Side=Right
  n : PMIOPort  Port=8  Side=Right
  connections:
  Pi Section Line/LConn1 -- N/RConn1
  Pi Section Line/RConn1 -- n/RConn1
  C/RConn1 -- Three-Phase PI Section Line/LConn3
  B/RConn1 -- Three-Phase PI Section Line/LConn2
  A/RConn1 -- Three-Phase PI Section Line/LConn1
  Three-Phase PI Section Line/RConn3 -- c/RConn1
  Three-Phase PI Section Line/RConn2 -- b/RConn1
  Three-Phase PI Section Line/RConn1 -- a/RConn1

== system LV_grid/L28/L1 ==
  Pi Section Line : powerlib/Elements/Pi Section Line  LConnTagsString=__new0  RConnTagsString=__new0  Frequency=50  Resistance=0.274  Inductance=0.073  Capacitance=12.74e-9  Length=0.0025  PiSections=1  Measurements=None
      settings: AttributesFormatString=\n  SourceProductName=Simscape Electrical  SourceProductBaseCode=PS
  Three-Phase PI Section Line : powerlib/Elements/Three-Phase PI Section Line  LConnTagsString=a|b|c  RConnTagsString=A|B|C  Frequency=50  Resistances=[ 0.274 0.959]  Inductances=[ 0.073 0.079]  Capacitances=[12.74e-9 7.751e-9]  Length=0.0025
      settings: SourceProductName=Simscape Electrical
  A : PMIOPort  Side=Left
  B : PMIOPort  Port=2  Side=Left
  C : PMIOPort  Port=3  Side=Left
  N : PMIOPort  Port=4  Side=Left
  a : PMIOPort  Port=5  Side=Right
  b : PMIOPort  Port=6  Side=Right
  c : PMIOPort  Port=7  Side=Right
  n : PMIOPort  Port=8  Side=Right
  connections:
  Pi Section Line/LConn1 -- N/RConn1
  Pi Section Line/RConn1 -- n/RConn1
  C/RConn1 -- Three-Phase PI Section Line/LConn3
  B/RConn1 -- Three-Phase PI Section Line/LConn2
  A/RConn1 -- Three-Phase PI Section Line/LConn1
  Three-Phase PI Section Line/RConn3 -- c/RConn1
  Three-Phase PI Section Line/RConn2 -- b/RConn1
  Three-Phase PI Section Line/RConn1 -- a/RConn1

== system LV_grid/L28/L2 ==
  Pi Section Line : powerlib/Elements/Pi Section Line  LConnTagsString=__new0  RConnTagsString=__new0  Frequency=50  Resistance=0.274  Inductance=0.073  Capacitance=12.74e-9  Length=0.0025  PiSections=1  Measurements=None
      settings: AttributesFormatString=\n  SourceProductName=Simscape Electrical  SourceProductBaseCode=PS
  Three-Phase PI Section Line : powerlib/Elements/Three-Phase PI Section Line  LConnTagsString=a|b|c  RConnTagsString=A|B|C  Frequency=50  Resistances=[ 0.274 0.959]  Inductances=[ 0.073 0.079]  Capacitances=[12.74e-9 7.751e-9]  Length=0.0025
      settings: SourceProductName=Simscape Electrical
  A : PMIOPort  Side=Left
  B : PMIOPort  Port=2  Side=Left
  C : PMIOPort  Port=3  Side=Left
  N : PMIOPort  Port=4  Side=Left
  a : PMIOPort  Port=5  Side=Right
  b : PMIOPort  Port=6  Side=Right
  c : PMIOPort  Port=7  Side=Right
  n : PMIOPort  Port=8  Side=Right
  connections:
  Pi Section Line/LConn1 -- N/RConn1
  Pi Section Line/RConn1 -- n/RConn1
  C/RConn1 -- Three-Phase PI Section Line/LConn3
  B/RConn1 -- Three-Phase PI Section Line/LConn2
  A/RConn1 -- Three-Phase PI Section Line/LConn1
  Three-Phase PI Section Line/RConn3 -- c/RConn1
  Three-Phase PI Section Line/RConn2 -- b/RConn1
  Three-Phase PI Section Line/RConn1 -- a/RConn1

== system LV_grid/L28/L3 ==
  Pi Section Line : powerlib/Elements/Pi Section Line  LConnTagsString=__new0  RConnTagsString=__new0  Frequency=50  Resistance=0.274  Inductance=0.073  Capacitance=12.74e-9  Length=0.0025  PiSections=1  Measurements=None
      settings: AttributesFormatString=\n  SourceProductName=Simscape Electrical  SourceProductBaseCode=PS
  Three-Phase PI Section Line : powerlib/Elements/Three-Phase PI Section Line  LConnTagsString=a|b|c  RConnTagsString=A|B|C  Frequency=50  Resistances=[ 0.274 0.959]  Inductances=[ 0.073 0.079]  Capacitances=[12.74e-9 7.751e-9]  Length=0.0025
      settings: SourceProductName=Simscape Electrical
  A : PMIOPort  Side=Left
  B : PMIOPort  Port=2  Side=Left
  C : PMIOPort  Port=3  Side=Left
  N : PMIOPort  Port=4  Side=Left
  a : PMIOPort  Port=5  Side=Right
  b : PMIOPort  Port=6  Side=Right
  c : PMIOPort  Port=7  Side=Right
  n : PMIOPort  Port=8  Side=Right
  connections:
  Pi Section Line/LConn1 -- N/RConn1
  Pi Section Line/RConn1 -- n/RConn1
  C/RConn1 -- Three-Phase PI Section Line/LConn3
  B/RConn1 -- Three-Phase PI Section Line/LConn2
  A/RConn1 -- Three-Phase PI Section Line/LConn1
  Three-Phase PI Section Line/RConn3 -- c/RConn1
  Three-Phase PI Section Line/RConn2 -- b/RConn1
  Three-Phase PI Section Line/RConn1 -- a/RConn1

== system LV_grid/L28/L4 ==
  Pi Section Line : powerlib/Elements/Pi Section Line  LConnTagsString=__new0  RConnTagsString=__new0  Frequency=50  Resistance=0.274  Inductance=0.073  Capacitance=12.74e-9  Length=0.0025  PiSections=1  Measurements=None
      settings: AttributesFormatString=\n  SourceProductName=Simscape Electrical  SourceProductBaseCode=PS
  Three-Phase PI Section Line : powerlib/Elements/Three-Phase PI Section Line  LConnTagsString=a|b|c  RConnTagsString=A|B|C  Frequency=50  Resistances=[ 0.274 0.959]  Inductances=[ 0.073 0.079]  Capacitances=[12.74e-9 7.751e-9]  Length=0.0025
      settings: SourceProductName=Simscape Electrical
  A : PMIOPort  Side=Left
  B : PMIOPort  Port=2  Side=Left
  C : PMIOPort  Port=3  Side=Left
  N : PMIOPort  Port=4  Side=Left
  a : PMIOPort  Port=5  Side=Right
  b : PMIOPort  Port=6  Side=Right
  c : PMIOPort  Port=7  Side=Right
  n : PMIOPort  Port=8  Side=Right
  connections:
  Pi Section Line/LConn1 -- N/RConn1
  Pi Section Line/RConn1 -- n/RConn1
  C/RConn1 -- Three-Phase PI Section Line/LConn3
  B/RConn1 -- Three-Phase PI Section Line/LConn2
  A/RConn1 -- Three-Phase PI Section Line/LConn1
  Three-Phase PI Section Line/RConn3 -- c/RConn1
  Three-Phase PI Section Line/RConn2 -- b/RConn1
  Three-Phase PI Section Line/RConn1 -- a/RConn1

== system LV_grid/L28/L5 ==
  Pi Section Line : powerlib/Elements/Pi Section Line  LConnTagsString=__new0  RConnTagsString=__new0  Frequency=50  Resistance=0.274  Inductance=0.073  Capacitance=12.74e-9  Length=0.0025  PiSections=1  Measurements=None
      settings: AttributesFormatString=\n  SourceProductName=Simscape Electrical  SourceProductBaseCode=PS
  Three-Phase PI Section Line : powerlib/Elements/Three-Phase PI Section Line  LConnTagsString=a|b|c  RConnTagsString=A|B|C  Frequency=50  Resistances=[ 0.274 0.959]  Inductances=[ 0.073 0.079]  Capacitances=[12.74e-9 7.751e-9]  Length=0.0025
      settings: SourceProductName=Simscape Electrical
  A : PMIOPort  Side=Left
  B : PMIOPort  Port=2  Side=Left
  C : PMIOPort  Port=3  Side=Left
  N : PMIOPort  Port=4  Side=Left
  a : PMIOPort  Port=5  Side=Right
  b : PMIOPort  Port=6  Side=Right
  c : PMIOPort  Port=7  Side=Right
  n : PMIOPort  Port=8  Side=Right
  connections:
  Pi Section Line/LConn1 -- N/RConn1
  Pi Section Line/RConn1 -- n/RConn1
  C/RConn1 -- Three-Phase PI Section Line/LConn3
  B/RConn1 -- Three-Phase PI Section Line/LConn2
  A/RConn1 -- Three-Phase PI Section Line/LConn1
  Three-Phase PI Section Line/RConn3 -- c/RConn1
  Three-Phase PI Section Line/RConn2 -- b/RConn1
  Three-Phase PI Section Line/RConn1 -- a/RConn1

== system LV_grid/L29/L1 ==
  Pi Section Line : powerlib/Elements/Pi Section Line  LConnTagsString=__new0  RConnTagsString=__new0  Frequency=50  Resistance=0.274  Inductance=0.073  Capacitance=12.74e-9  Length=0.0025  PiSections=1  Measurements=None
      settings: AttributesFormatString=\n  SourceProductName=Simscape Electrical  SourceProductBaseCode=PS
  Three-Phase PI Section Line : powerlib/Elements/Three-Phase PI Section Line  LConnTagsString=a|b|c  RConnTagsString=A|B|C  Frequency=50  Resistances=[ 0.274 0.959]  Inductances=[ 0.073 0.079]  Capacitances=[12.74e-9 7.751e-9]  Length=0.0025
      settings: SourceProductName=Simscape Electrical
  A : PMIOPort  Side=Left
  B : PMIOPort  Port=2  Side=Left
  C : PMIOPort  Port=3  Side=Left
  N : PMIOPort  Port=4  Side=Left
  a : PMIOPort  Port=5  Side=Right
  b : PMIOPort  Port=6  Side=Right
  c : PMIOPort  Port=7  Side=Right
  n : PMIOPort  Port=8  Side=Right
  connections:
  Pi Section Line/LConn1 -- N/RConn1
  Pi Section Line/RConn1 -- n/RConn1
  C/RConn1 -- Three-Phase PI Section Line/LConn3
  B/RConn1 -- Three-Phase PI Section Line/LConn2
  A/RConn1 -- Three-Phase PI Section Line/LConn1
  Three-Phase PI Section Line/RConn3 -- c/RConn1
  Three-Phase PI Section Line/RConn2 -- b/RConn1
  Three-Phase PI Section Line/RConn1 -- a/RConn1

== system LV_grid/L29/L2 ==
  Pi Section Line : powerlib/Elements/Pi Section Line  LConnTagsString=__new0  RConnTagsString=__new0  Frequency=50  Resistance=0.274  Inductance=0.073  Capacitance=12.74e-9  Length=0.0025  PiSections=1  Measurements=None
      settings: AttributesFormatString=\n  SourceProductName=Simscape Electrical  SourceProductBaseCode=PS
  Three-Phase PI Section Line : powerlib/Elements/Three-Phase PI Section Line  LConnTagsString=a|b|c  RConnTagsString=A|B|C  Frequency=50  Resistances=[ 0.274 0.959]  Inductances=[ 0.073 0.079]  Capacitances=[12.74e-9 7.751e-9]  Length=0.0025
      settings: SourceProductName=Simscape Electrical
  A : PMIOPort  Side=Left
  B : PMIOPort  Port=2  Side=Left
  C : PMIOPort  Port=3  Side=Left
  N : PMIOPort  Port=4  Side=Left
  a : PMIOPort  Port=5  Side=Right
  b : PMIOPort  Port=6  Side=Right
  c : PMIOPort  Port=7  Side=Right
  n : PMIOPort  Port=8  Side=Right
  connections:
  Pi Section Line/LConn1 -- N/RConn1
  Pi Section Line/RConn1 -- n/RConn1
  C/RConn1 -- Three-Phase PI Section Line/LConn3
  B/RConn1 -- Three-Phase PI Section Line/LConn2
  A/RConn1 -- Three-Phase PI Section Line/LConn1
  Three-Phase PI Section Line/RConn3 -- c/RConn1
  Three-Phase PI Section Line/RConn2 -- b/RConn1
  Three-Phase PI Section Line/RConn1 -- a/RConn1

== system LV_grid/L29/L3 ==
  Pi Section Line : powerlib/Elements/Pi Section Line  LConnTagsString=__new0  RConnTagsString=__new0  Frequency=50  Resistance=0.274  Inductance=0.073  Capacitance=12.74e-9  Length=0.0025  PiSections=1  Measurements=None
      settings: AttributesFormatString=\n  SourceProductName=Simscape Electrical  SourceProductBaseCode=PS
  Three-Phase PI Section Line : powerlib/Elements/Three-Phase PI Section Line  LConnTagsString=a|b|c  RConnTagsString=A|B|C  Frequency=50  Resistances=[ 0.274 0.959]  Inductances=[ 0.073 0.079]  Capacitances=[12.74e-9 7.751e-9]  Length=0.0025
      settings: SourceProductName=Simscape Electrical
  A : PMIOPort  Side=Left
  B : PMIOPort  Port=2  Side=Left
  C : PMIOPort  Port=3  Side=Left
  N : PMIOPort  Port=4  Side=Left
  a : PMIOPort  Port=5  Side=Right
  b : PMIOPort  Port=6  Side=Right
  c : PMIOPort  Port=7  Side=Right
  n : PMIOPort  Port=8  Side=Right
  connections:
  Pi Section Line/LConn1 -- N/RConn1
  Pi Section Line/RConn1 -- n/RConn1
  C/RConn1 -- Three-Phase PI Section Line/LConn3
  B/RConn1 -- Three-Phase PI Section Line/LConn2
  A/RConn1 -- Three-Phase PI Section Line/LConn1
  Three-Phase PI Section Line/RConn3 -- c/RConn1
  Three-Phase PI Section Line/RConn2 -- b/RConn1
  Three-Phase PI Section Line/RConn1 -- a/RConn1

== system LV_grid/L29/L4 ==
  Pi Section Line : powerlib/Elements/Pi Section Line  LConnTagsString=__new0  RConnTagsString=__new0  Frequency=50  Resistance=0.274  Inductance=0.073  Capacitance=12.74e-9  Length=0.0025  PiSections=1  Measurements=None
      settings: AttributesFormatString=\n  SourceProductName=Simscape Electrical  SourceProductBaseCode=PS
  Three-Phase PI Section Line : powerlib/Elements/Three-Phase PI Section Line  LConnTagsString=a|b|c  RConnTagsString=A|B|C  Frequency=50  Resistances=[ 0.274 0.959]  Inductances=[ 0.073 0.079]  Capacitances=[12.74e-9 7.751e-9]  Length=0.0025
      settings: SourceProductName=Simscape Electrical
  A : PMIOPort  Side=Left
  B : PMIOPort  Port=2  Side=Left
  C : PMIOPort  Port=3  Side=Left
  N : PMIOPort  Port=4  Side=Left
  a : PMIOPort  Port=5  Side=Right
  b : PMIOPort  Port=6  Side=Right
  c : PMIOPort  Port=7  Side=Right
  n : PMIOPort  Port=8  Side=Right
  connections:
  Pi Section Line/LConn1 -- N/RConn1
  Pi Section Line/RConn1 -- n/RConn1
  C/RConn1 -- Three-Phase PI Section Line/LConn3
  B/RConn1 -- Three-Phase PI Section Line/LConn2
  A/RConn1 -- Three-Phase PI Section Line/LConn1
  Three-Phase PI Section Line/RConn3 -- c/RConn1
  Three-Phase PI Section Line/RConn2 -- b/RConn1
  Three-Phase PI Section Line/RConn1 -- a/RConn1

== system LV_grid/L29/L5 ==
  Pi Section Line : powerlib/Elements/Pi Section Line  LConnTagsString=__new0  RConnTagsString=__new0  Frequency=50  Resistance=0.274  Inductance=0.073  Capacitance=12.74e-9  Length=0.0025  PiSections=1  Measurements=None
      settings: AttributesFormatString=\n  SourceProductName=Simscape Electrical  SourceProductBaseCode=PS
  Three-Phase PI Section Line : powerlib/Elements/Three-Phase PI Section Line  LConnTagsString=a|b|c  RConnTagsString=A|B|C  Frequency=50  Resistances=[ 0.274 0.959]  Inductances=[ 0.073 0.079]  Capacitances=[12.74e-9 7.751e-9]  Length=0.0025
      settings: SourceProductName=Simscape Electrical
  A : PMIOPort  Side=Left
  B : PMIOPort  Port=2  Side=Left
  C : PMIOPort  Port=3  Side=Left
  N : PMIOPort  Port=4  Side=Left
  a : PMIOPort  Port=5  Side=Right
  b : PMIOPort  Port=6  Side=Right
  c : PMIOPort  Port=7  Side=Right
  n : PMIOPort  Port=8  Side=Right
  connections:
  Pi Section Line/LConn1 -- N/RConn1
  Pi Section Line/RConn1 -- n/RConn1
  C/RConn1 -- Three-Phase PI Section Line/LConn3
  B/RConn1 -- Three-Phase PI Section Line/LConn2
  A/RConn1 -- Three-Phase PI Section Line/LConn1
  Three-Phase PI Section Line/RConn3 -- c/RConn1
  Three-Phase PI Section Line/RConn2 -- b/RConn1
  Three-Phase PI Section Line/RConn1 -- a/RConn1
